simulink model "noTopLevelStates"  (Simulink 7.6)
settings: Solver=FixedStepDiscrete  StartTime=0.0  StopTime=10.0  FixedStep=1  RelTol=1e-3
settings Model: Creator=c2wt  LastModifiedBy=c2wt

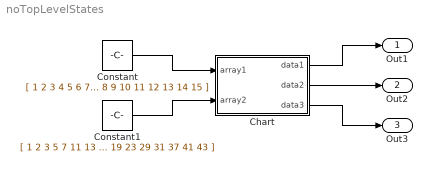
== system noTopLevelStates ==
  Chart : Stateflow chart  TreatAsAtomicUnit=on
  Constant : Constant  Value=[ 1 2 3 4 5 6 7 8 9 10 11 12 13 14 15 ]
  Constant1 : Constant  Value=[ 1 2 3 5 7 11 13 17 19 23 29 31 37 41 43 ]
  Out1 : Outport
  Out2 : Outport  Port=2
  Out3 : Outport  Port=3
  wires:
  Chart/1(data1) -> Out1/1
  Constant/1 -> Chart/1(array1)
  Constant1/1 -> Chart/2(array2)
  Chart/2(data2) -> Out2/1
  Chart/3(data3) -> Out3/1

== stateflow chart Chart ==
  (default) -> (junction 3)
  (junction 3) -> (junction 4) : { data1 = array2[ array1[ data ] - 1 ]; data2 = data;}
  (junction 4) -> (junction 5) : { data++; data3 = data; }
  data: data local double =0; data1 output double; array1 input double size=15; array2 input double size=15; data2 output double; data3 output double
